simulink model "LQR_obs"  (R2025b)
settings: Solver=VariableStepAuto  StartTime=0.0  StopTime=20  RelTol=1e-3
values from neighbouring files (symbols this model uses):
  A = [0 1 0 0;     (m_b*g*r^2)/(I_b*l) 0 (m_b*g*r^2)/(I_b) 0 ;      0 0 0 1;    20 0 (M_r*d*g)/I_r 0 ]    [Copy_of_LQR_ctrl.m]    (also in LQR_ctrl.m = [0 1 0 0;     A1(1,1) 0 A1(1,2) 0;     0 0 0 1;     A1(2,1) ; Rlocus_ctrl.m = [0 1 0 0;     A1(1,1) 0 A1(1,2) 0;     0 0 0 1;     A1(2,1) ; State4.m = [0 1 0 0;     A1(1,1) 0 A1(1,2) 0;     0 0 0 1;     A1(2,1) ; pole_placement_ctrl.m = [0 1 0 0;     A1(1,1) 0 A1(1,2) 0;     0 0 0 1;     A1(2,1) )
  B = -[0 ; 0; 0 ; ((I_w/R) + (M_w+M_r)*R)/(I_r)]    [Copy_of_LQR_ctrl.m]    (also in LQR_ctrl.m = -[0 ; B1(1); 0 ; B1(2)]; Rlocus_ctrl.m = -[0 ; B1(1); 0 ; B1(2)]; State4.m = -[0 ; B1(1); 0 ; B1(2)]; pole_placement_ctrl.m = -[0 ; B1(1); 0 ; B1(2)])
  C = [0 0 1 0]    [Copy_of_LQR_ctrl.m]    (also in LQR_ctrl.m; Rlocus_ctrl.m = eye(4); State4.m = eye(4); pole_placement_ctrl.m = eye(4))
  K = lqr(A, B, Q, R)    [LQR_ctrl.m]    (also in State4.m; pole_placement_ctrl.m = place(A,B,poles))
  Ke = L    [Copy_of_LQR_ctrl.m]    (also in LQR_ctrl.m)
  x0 = [0.01, 0, deg2rad(5),0]'    [Copy_of_LQR_ctrl.m]    (also in LQR_ctrl.m = [0.005, 0, -deg2rad(2),0]'; State4.m = x0 - x_ref; pole_placement_ctrl.m = [0.005;0;deg2rad(0);0])
  x0_o = [0.02;0;deg2rad(7.5);0]    [Copy_of_LQR_ctrl.m]    (also in LQR_ctrl.m = [-0.002;0;deg2rad(5);0])
settings Model: Creator=Abhi  LastModifiedBy=Abhi

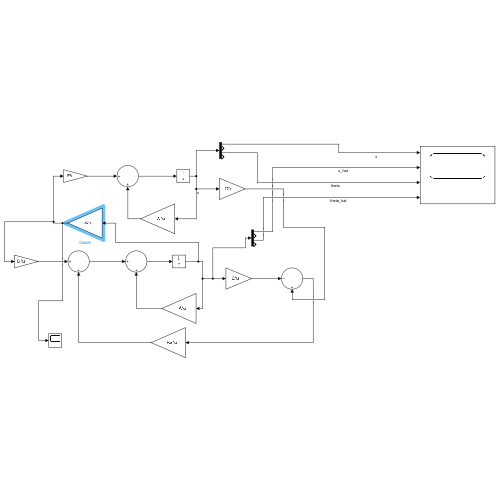
[thumbnail: Simulink's stored preview of the top-level diagram]
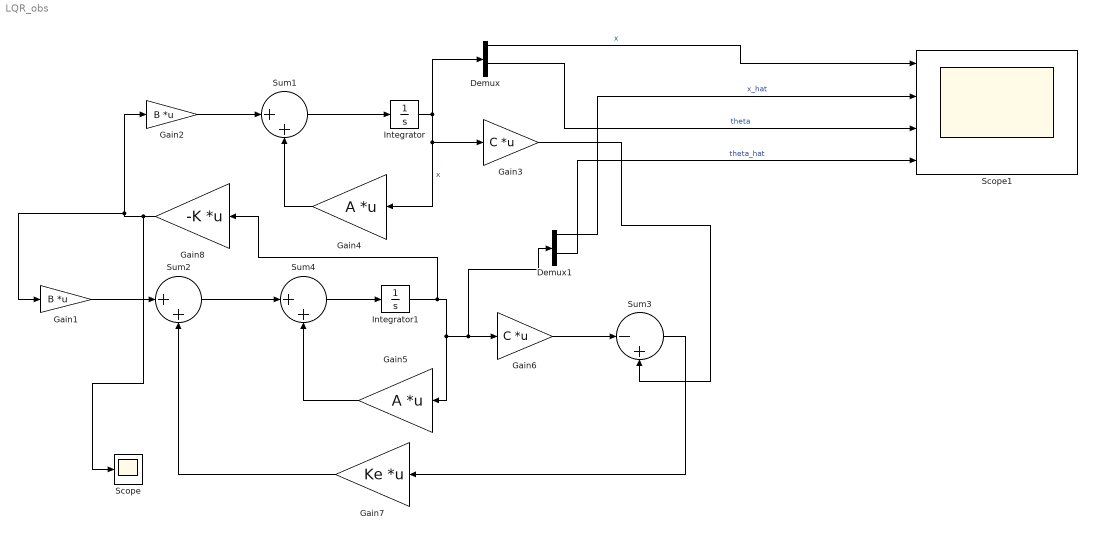
== system LQR_obs ==
  Demux : Demux
  Demux1 : Demux
  Gain1 : Gain  Gain=B  Multiplication=Matrix(K*u)
  Gain2 : Gain  Gain=B  Multiplication=Matrix(K*u)
  Gain3 : Gain  Gain=C  Multiplication=Matrix(K*u)
  Gain4 : Gain  Gain=A  Multiplication=Matrix(K*u)
  Gain5 : Gain  Gain=A  Multiplication=Matrix(K*u)
  Gain6 : Gain  Gain=C  Multiplication=Matrix(K*u)
  Gain7 : Gain  Gain=Ke  Multiplication=Matrix(K*u)
  Gain8 : Gain  Gain=-K  Multiplication=Matrix(K*u)
  Integrator : Integrator  InitialCondition=x0
  Integrator1 : Integrator  InitialCondition=x0_o
  Scope : Scope
      settings: ActiveDisplayYMinimum=-130.02247832697481  ActiveDisplayYMaximum=15.739943039239076
  Scope1 : Scope  NumInputPorts=4
      settings: SampleTime=1e-4  ActiveDisplayYMinimum=-0.11223368726657734  ActiveDisplayYMaximum=0.025910198708945818
  Sum1 : Sum  Inputs=|++
  Sum2 : Sum  Inputs=|++
  Sum3 : Sum  Inputs=|-+
  Sum4 : Sum  Inputs=|++
  wires:
  Sum1/1 -> Integrator/1
  Gain3/1 -> Sum3/2
  Gain4/1 -> Sum1/2
  Gain2/1 -> Sum1/1
  Gain1/1 -> Sum2/1
  Integrator/1 -> Gain3/1, Gain4/1, Demux/1  "x"
  Sum3/1 -> Gain7/1
  Integrator1/1 -> Gain8/1, Demux1/1, Gain6/1, Gain5/1
  Gain6/1 -> Sum3/1
  Gain5/1 -> Sum4/2
  Sum2/1 -> Sum4/1
  Sum4/1 -> Integrator1/1
  Gain7/1 -> Sum2/2
  Gain8/1 -> Scope/1, Gain1/1, Gain2/1
  Demux1/1 -> Scope1/2  "x_hat"
  Demux1/3 -> Scope1/4  "theta_hat"
  Demux/3 -> Scope1/3  "theta"
  Demux/1 -> Scope1/1  "x"
